simulink model "pole_placement"  (R2017a)
settings: Solver=VariableStepAuto  StartTime=0.0  StopTime=5  RelTol=1e-3
values from neighbouring files (symbols this model uses):
  DCgain5 = D5d + C5cl*inv(eye(3)-A5cl)*B5d    [q13.m]    (also in q5.m; q5_reduced.m)
  h5 = 2.5*pi/w    [q13.m]    (also in q5.m = 2*pi/w; q5_reduced.m = 2*pi/w)
  K5_discr = place(A5d, B5d, P_discr)    [q13.m]    (also in q5.m; q5_reduced.m)
undefined symbols (not defined in the file or in its folder): A5d, B5d, C5d, D5d
settings Model: Creator=Aleksandra  LastModifiedBy=Aleksandra

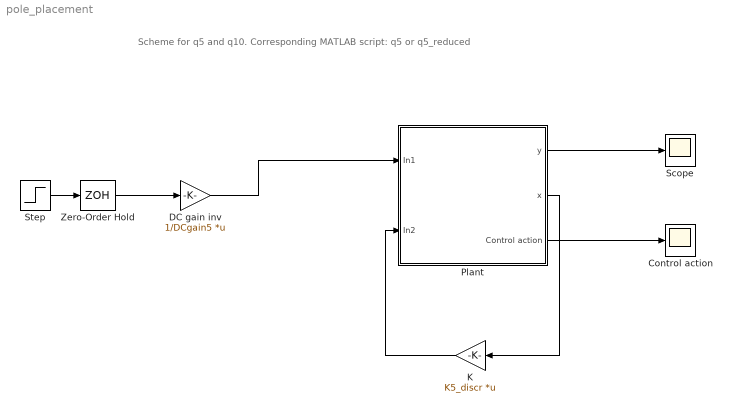
== system pole_placement ==
  note: Scheme for q5 and q10.
      | Corresponding MATLAB script: q5 or q5_reduced
  Control action : Scope
  DC gain inv : Gain  Gain=1/DCgain5  Multiplication=Matrix(K*u)
  K : Gain  Gain=K5_discr  Multiplication=Matrix(K*u)
  Plant : Subsystem
  Scope : Scope
  Step : Step  Time=0  SampleTime=0
  Zero-Order Hold : ZeroOrderHold  SampleTime=h5
  wires:
  Step/1 -> Zero-Order Hold/1
  Plant/1(y) -> Scope/1
  Plant/2(x) -> K/1
  K/1 -> Plant/2(In2)
  Plant/3(Control action) -> Control action/1
  Zero-Order Hold/1 -> DC gain inv/1
  DC gain inv/1 -> Plant/1(In1)

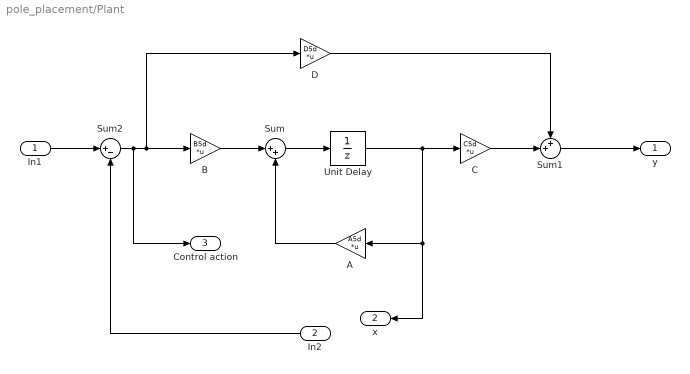
== system pole_placement/Plant ==
  In1 : Inport
  In2 : Inport  Port=2
  A : Gain  Gain=A5d  Multiplication=Matrix(K*u)
  B : Gain  Gain=B5d  Multiplication=Matrix(K*u)
  C : Gain  Gain=C5d  Multiplication=Matrix(K*u)
  D : Gain  Gain=D5d  Multiplication=Matrix(K*u)
  Sum : Sum  Inputs=|++
  Sum1 : Sum  Inputs=++|
  Sum2 : Sum  Inputs=|+-
  Unit Delay : UnitDelay  SampleTime=-1
  y : Outport
  x : Outport  Port=2
  Control action : Outport  Port=3
  wires:
  Sum/1 -> Unit Delay/1
  A/1 -> Sum/2
  D/1 -> Sum1/1
  C/1 -> Sum1/2
  Sum1/1 -> y/1
  B/1 -> Sum/1
  Sum2/1 -> Control action/1, D/1, B/1
  Unit Delay/1 -> x/1, A/1, C/1
  In2/1 -> Sum2/2
  In1/1 -> Sum2/1
